simulink model "m20220211_2_fixedDynaModel_varParams_2"  (R2021b)
settings: Solver=ode15s  StartTime=0.0  StopTime=2749  FixedStep=1/33  MaxStep=.1  RelTol=1e-3  AbsTol=1e-3  EnableMultiTasking=on
undefined symbols (not defined in the file or in its folder): f3SecFixedDyna_mex, fkin_3sec_tips_mex
settings Model: Creator=isuru  LastModifiedBy=Dulanjana
settings SolverCC: AutoScaleAbsTol=off  ExtrapolationOrder=1  AlgebraicLoopSolver=TrustRegion
settings DataIOCC: LimitDataPoints=on  SaveFormat=Array  ReturnWorkspaceOutputs=off
settings OptimizationCC: LifeSpan=inf
settings DebuggingCC: UnderspecifiedInitializationDetection=Classic  MergeDetectMultiDrivingBlocksExec=none  SolverPrmCheckMsg=warning  StateNameClashWarn=warning  SFUnexpectedBacktrackingDiag=warning  SFNoUnconditionalDefaultTransitionDiag=warning  SFExecutionAtInitializationDiag=none  SFMachineParentedDataDiag=warning  ArithmeticOperatorsInVariantConditions=warning
settings HardwareCC: ProdBitPerPointer=32  ProdBitPerSizeT=32  ProdBitPerPtrDiffT=32  ProdLargestAtomicFloat=None  ProdIntDivRoundTo=Undefined  ProdEndianess=Unspecified  ProdWordSize=32  ProdHWDeviceType=32-bit Generic
settings ModelReferenceCC: PropagateSignalLabelsOutOfModel=off
settings SFSimCC: SimUseLocalCustomCode=off  CustomCodeUndefinedFunction=UseInterfaceOnly
settings RTWCC: RTWUseLocalCustomCode=off
settings CodeAppCC: StateflowObjectComments=on
settings GRTTargetCC: TargetLangStandard=C89/C90 (ANSI)
settings ConfigComp: CovMetricSettings=dw  CovSaveCumulativeToWorkspaceVar=on  CovSaveSingleToWorkspaceVar=on  CovExternalEMLEnable=off  CovSFcnEnable=off

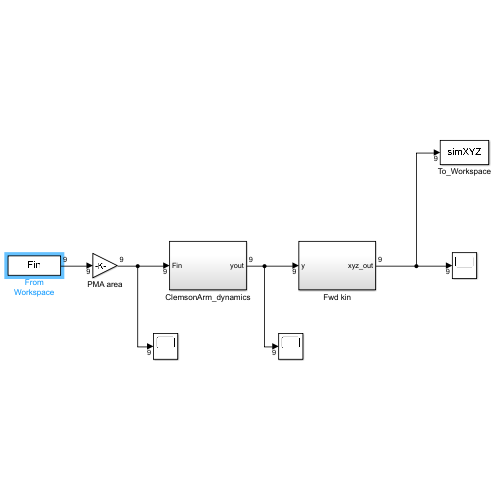
[thumbnail: Simulink's stored preview of the top-level diagram]
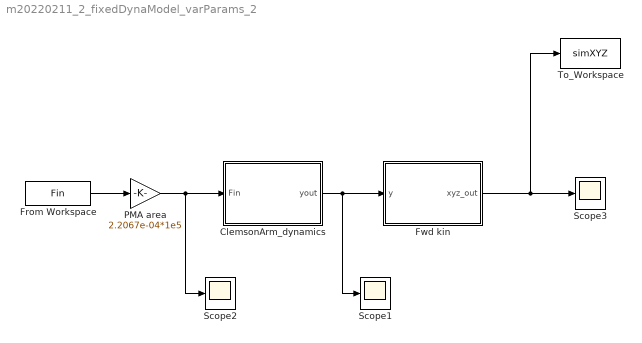
== system m20220211_2_fixedDynaModel_varParams_2 ==
  ClemsonArm_dynamics : Subsystem
  From Workspace : FromWorkspace  VariableName=Fin  SampleTime=-1  Interpolate=off  OutputAfterFinalValue=Holding final value
  Fwd kin : Subsystem
  PMA area : Gain  Gain=2.2067e-04*1e5
  Scope1 : Scope
  Scope2 : Scope
  Scope3 : Scope
  To_Workspace : ToWorkspace  VariableName=simXYZ  SaveFormat=Timeseries  SampleTime=0.05
  wires:
  ClemsonArm_dynamics/1(yout) -> Scope1/1, Fwd kin/1(y)
  From Workspace/1 -> PMA area/1
  PMA area/1 -> Scope2/1, ClemsonArm_dynamics/1(Fin)
  Fwd kin/1(xyz_out) -> Scope3/1, To_Workspace/1

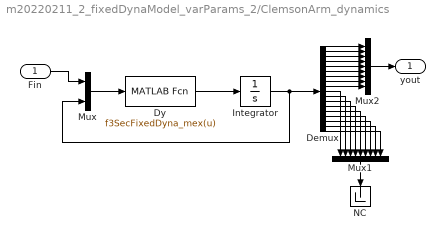
== system m20220211_2_fixedDynaModel_varParams_2/ClemsonArm_dynamics ==
  Fin : Inport
  Demux : Demux  Outputs=18
  Dy : MATLABFcn  MATLABFcn=f3SecFixedDyna_mex(u)
  Integrator : Integrator  InitialCondition=[0 0 0 0 0 0 0 0 0 0 0 0 0 0 0 0 0 0]
  Mux : Mux  Inputs=2
  Mux1 : Mux  Inputs=9
  Mux2 : Mux  Inputs=9
  NC : Terminator
  yout : Outport  VectorParamsAs1DForOutWhenUnconnected=off
  wires:
  Dy/1 -> Integrator/1
  Demux/6 -> Mux2/6
  Demux/5 -> Mux2/5
  Integrator/1 -> Mux/2, Demux/1
  Demux/9 -> Mux2/9
  Demux/4 -> Mux2/4
  Demux/2 -> Mux2/2
  Demux/1 -> Mux2/1
  Mux1/1 -> NC/1
  Mux2/1 -> yout/1
  Fin/1 -> Mux/1
  Demux/3 -> Mux2/3
  Demux/7 -> Mux2/7
  Demux/11 -> Mux1/2
  Demux/17 -> Mux1/8
  Demux/10 -> Mux1/1
  Demux/12 -> Mux1/3
  Demux/15 -> Mux1/6
  Mux/1 -> Dy/1
  Demux/18 -> Mux1/9
  Demux/14 -> Mux1/5
  Demux/8 -> Mux2/8
  Demux/16 -> Mux1/7
  Demux/13 -> Mux1/4

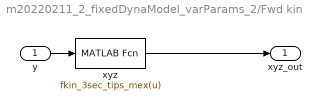
== system m20220211_2_fixedDynaModel_varParams_2/Fwd kin ==
  y : Inport
  xyz : MATLABFcn  MATLABFcn=fkin_3sec_tips_mex(u)
  xyz_out : Outport  VectorParamsAs1DForOutWhenUnconnected=off
  wires:
  y/1 -> xyz/1
  xyz/1 -> xyz_out/1
